simulink model "simple_stateflow"  (R2024b)
settings: Solver=ode3  StartTime=0.0  StopTime=20.0  FixedStep=0.1  RelTol=1e-3
settings Model: Creator=balaj  LastModifiedBy=balaj

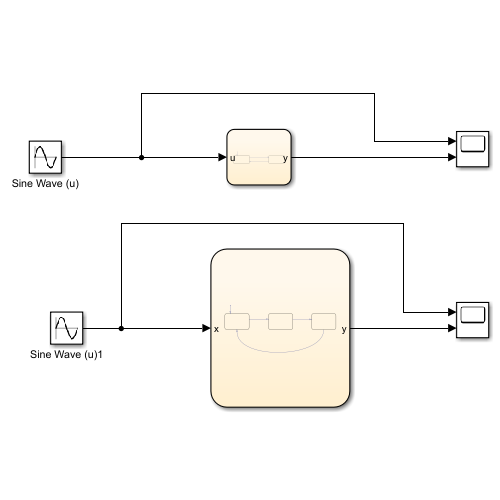
[thumbnail: Simulink's stored preview of the top-level diagram]
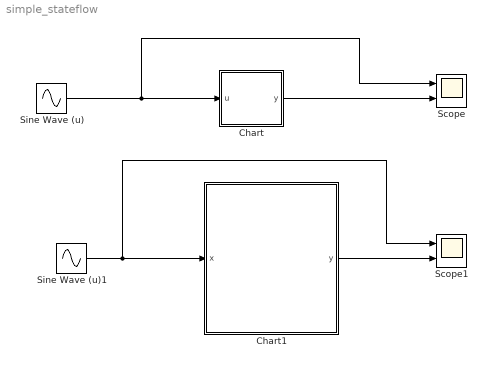
== system simple_stateflow ==
  Chart : Stateflow chart  TreatAsAtomicUnit=on
  Chart1 : Stateflow chart  TreatAsAtomicUnit=on
  Scope : Scope  NumInputPorts=2
  Scope1 : Scope  NumInputPorts=2
  Sine Wave (u) : Sin  SampleTime=0
  Sine Wave (u)1 : Sin  SampleTime=0
  wires:
  Sine Wave (u)/1 -> Scope/1, Chart/1(u)
  Chart/1(y) -> Scope/2
  Sine Wave (u)1/1 -> Scope1/1, Chart1/1(x)
  Chart1/1(y) -> Scope1/2

== stateflow chart simple_stateflow/Chart1 ==
  state State1
    y=10;
  state State2
    y=3;
  state State3
    y=2;
  (default) -> State1
  State1 -> State2 : [x<0]
  State2 -> State3 : [x>0]
  State3 -> State1 : [x==0]
  data: x input; y output

== stateflow chart simple_stateflow/Chart ==
  state ON
    y=1;
  state OFF
    y=-1;
  (default) -> ON
  ON -> OFF : [u<0]
  OFF -> ON : [u>0]
  data: u input; y output
